simulink model "half_total_adder"  (R2018a)
settings: Solver=VariableStepAuto  StartTime=0.0  StopTime=10.0  RelTol=1e-3
settings Model: Creator=Edoardo Debenedetti  LastModifiedBy=Edoardo Debenedetti

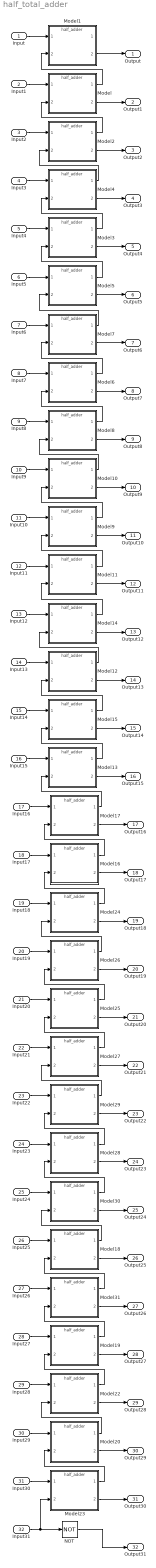
== system half_total_adder ==
  Input : Inport
  Input1 : Inport  Port=2
  Input2 : Inport  Port=3
  Input3 : Inport  Port=4
  Input4 : Inport  Port=5
  Input5 : Inport  Port=6
  Input6 : Inport  Port=7
  Input7 : Inport  Port=8
  Input8 : Inport  Port=9
  Input9 : Inport  Port=10
  Input10 : Inport  Port=11
  Input11 : Inport  Port=12
  Input12 : Inport  Port=13
  Input13 : Inport  Port=14
  Input14 : Inport  Port=15
  Input15 : Inport  Port=16
  Input16 : Inport  Port=17
  Input17 : Inport  Port=18
  Input18 : Inport  Port=19
  Input19 : Inport  Port=20
  Input20 : Inport  Port=21
  Input21 : Inport  Port=22
  Input22 : Inport  Port=23
  Input23 : Inport  Port=24
  Input24 : Inport  Port=25
  Input25 : Inport  Port=26
  Input26 : Inport  Port=27
  Input27 : Inport  Port=28
  Input28 : Inport  Port=29
  Input29 : Inport  Port=30
  Input30 : Inport  Port=31
  Input31 : Inport  Port=32
  Model{,1..20,22..31} (31 alike) : ModelReference  ModelNameDialog=half_adder  SimulationMode=Normal  ModelReferenceVersion=1.2
  NOT : Logic  Operator=NOT  IconShape=distinctive  AllPortsSameDT=off  OutDataTypeStr=boolean
  Output : Outport
  Output1 : Outport  Port=2
  Output2 : Outport  Port=3
  Output3 : Outport  Port=4
  Output4 : Outport  Port=5
  Output5 : Outport  Port=6
  Output6 : Outport  Port=7
  Output7 : Outport  Port=8
  Output8 : Outport  Port=9
  Output9 : Outport  Port=10
  Output10 : Outport  Port=11
  Output11 : Outport  Port=12
  Output12 : Outport  Port=13
  Output13 : Outport  Port=14
  Output14 : Outport  Port=15
  Output15 : Outport  Port=16
  Output16 : Outport  Port=17
  Output17 : Outport  Port=18
  Output18 : Outport  Port=19
  Output19 : Outport  Port=20
  Output20 : Outport  Port=21
  Output21 : Outport  Port=22
  Output22 : Outport  Port=23
  Output23 : Outport  Port=24
  Output24 : Outport  Port=25
  Output25 : Outport  Port=26
  Output26 : Outport  Port=27
  Output27 : Outport  Port=28
  Output28 : Outport  Port=29
  Output29 : Outport  Port=30
  Output30 : Outport  Port=31
  Output31 : Outport  Port=32
  wires:
  Input1/1 -> Model/1
  Model/1 -> Model1/2
  Input/1 -> Model1/1
  Model1/2 -> Output/1
  Model/2 -> Output1/1
  Model2/2 -> Output2/1
  Model2/1 -> Model/2
  Input2/1 -> Model2/1
  Model4/1 -> Model2/2
  Input5/1 -> Model5/1
  Model5/1 -> Model3/2
  Model5/2 -> Output5/1
  Model3/2 -> Output4/1
  Model4/2 -> Output3/1
  Input3/1 -> Model4/1
  Model3/1 -> Model4/2
  Input4/1 -> Model3/1
  Input10/1 -> Model9/1
  Model9/1 -> Model10/2
  Input9/1 -> Model10/1
  Model10/2 -> Output9/1
  Model9/2 -> Output10/1
  Model11/2 -> Output11/1
  Model11/1 -> Model9/2
  Input11/1 -> Model11/1
  Model10/1 -> Model8/2
  Model7/1 -> Model5/2
  Input8/1 -> Model8/1
  Model8/1 -> Model6/2
  Model8/2 -> Output8/1
  Model6/2 -> Output7/1
  Model7/2 -> Output6/1
  Input6/1 -> Model7/1
  Model6/1 -> Model7/2
  Input7/1 -> Model6/1
  Model14/2 -> Output12/1
  Model14/1 -> Model11/2
  Input12/1 -> Model14/1
  Model12/1 -> Model14/2
  Input15/1 -> Model13/1
  Model13/1 -> Model15/2
  Model13/2 -> Output15/1
  Model15/2 -> Output14/1
  Model12/2 -> Output13/1
  Input13/1 -> Model12/1
  Model15/1 -> Model12/2
  Input14/1 -> Model15/1
  Input30/1 -> Model23/1
  Model23/1 -> Model20/2
  Input29/1 -> Model20/1
  Model20/2 -> Output29/1
  Model23/2 -> Output30/1
  NOT/1 -> Output31/1
  Input31/1 -> NOT/1, Model23/2
  Model20/1 -> Model22/2
  Input28/1 -> Model22/1
  Model22/1 -> Model19/2
  Model22/2 -> Output28/1
  Input23/1 -> Model28/1
  Model28/1 -> Model29/2
  Input22/1 -> Model29/1
  Model29/2 -> Output22/1
  Model28/2 -> Output23/1
  Model30/2 -> Output24/1
  Model30/1 -> Model28/2
  Input24/1 -> Model30/1
  Model29/1 -> Model27/2
  Model18/1 -> Model30/2
  Input27/1 -> Model19/1
  Model19/1 -> Model31/2
  Model19/2 -> Output27/1
  Model31/2 -> Output26/1
  Model18/2 -> Output25/1
  Input25/1 -> Model18/1
  Model31/1 -> Model18/2
  Input26/1 -> Model31/1
  Input20/1 -> Model25/1
  Model25/1 -> Model26/2
  Input19/1 -> Model26/1
  Model26/2 -> Output19/1
  Model25/2 -> Output20/1
  Model27/2 -> Output21/1
  Model27/1 -> Model25/2
  Input21/1 -> Model27/1
  Model26/1 -> Model24/2
  Model17/1 -> Model13/2
  Input18/1 -> Model24/1
  Model24/1 -> Model16/2
  Model24/2 -> Output18/1
  Model16/2 -> Output17/1
  Model17/2 -> Output16/1
  Input16/1 -> Model17/1
  Model16/1 -> Model17/2
  Input17/1 -> Model16/1
